simulink model "pendulo_rueda_lazo_cerrado_LQR"  (R2021b)
settings: Solver=ode5  StartTime=0.0  StopTime=30  FixedStep=0.01  RelTol=1e-3  EnableMultiTasking=on
values from neighbouring files (symbols this model uses):
  A = [0, 1, 0, 0;b4, 0, 0, b5;0, 0, 0, 1;b7, 0, 0, b8]    [Diseno_controlador_LQR.m]
  B = [0;b6;0;b9]    [Diseno_controlador_LQR.m]
  C = [1,0,0,0;0,0,1,0]    [Diseno_controlador_LQR.m]
  K_LQR = lqr(A,B,Q,r)    [Diseno_controlador_LQR.m]
undefined symbols (not defined in the file or in its folder): Ke_uno, National_Instruments, PCIe
libraries: sldrtlib x5
Description:
  | Real-Time Van der Pol Simulation
  | 
  | The example model "sldrtex_vdp" shows a real-time version of the Simulink(R) Van der Pol
  | simulation model. This model does not need any external signals, so it does
  | not need any data acquisition hardware or driver. This makes the model ideal
  | for the first experiments with Simulink Desktop Real-Time(TM), without need to
  | worry about proper I/O hardware configuration.
  | 
  | How to run this model in Normal Mode:
  | 
  | 1) Double-click the orange button to switch to Normal Mode if needed.
  | 2) Start the real-time execution using Simulation->Run.
  | 3) Observe any missed ticks on the Missed Ticks scope.
  | 
  | How to run this model in External Mode:
  | 
  | 1) Double-click the orange button to switch to External Mode if needed.
  | 2) Start the real-time execution using Simulation->Run. The model will automatically
  |    build, connect to Simulink in External Mode and start.
  | 3) Missed ticks will be always zero.
settings Model: ExtModeTrigDuration=100001  ExtModeLogAll=off  Creator=The MathWorks, Inc.  LastModifiedBy=USUARIO
settings SolverCC: AlgebraicLoopSolver=TrustRegion
settings DataIOCC: LimitDataPoints=on  SaveFormat=Array  ReturnWorkspaceOutputs=off  SignalLoggingName=logsOut
settings OptimizationCC: ExpressionDepthLimit=2147483647  InitFltsAndDblsToZero=on  EfficientMapNaN2IntZero=off  LifeSpan=inf
settings DebuggingCC: UnderspecifiedInitializationDetection=Classic  MergeDetectMultiDrivingBlocksExec=none  SignalResolutionControl=TryResolveAllWithWarning  FcnCallInpInsideContextMsg=warning  AllowSymbolicDim=off  StateNameClashWarn=warning  SymbolicDimsDataTypeCodeGenerationDiagnostic=none  SFUnexpectedBacktrackingDiag=warning  SFNoUnconditionalDefaultTransitionDiag=warning  SFExecutionAtInitializationDiag=none  SFMachineParentedDataDiag=warning  ArithmeticOperatorsInVariantConditions=warning
settings HardwareCC: TargetBitPerLong=64  TargetBitPerPointer=64  TargetBitPerSizeT=64  TargetBitPerPtrDiffT=64  TargetIntDivRoundTo=Zero  TargetEndianess=LittleEndian  TargetWordSize=64  TargetHWDeviceType=Intel->x86-64
settings ModelReferenceCC: PropagateSignalLabelsOutOfModel=off
settings SFSimCC: SimUseLocalCustomCode=off
settings RTWCC: Description=Simulink Desktop Real-Time  SystemTargetFile=sldrt.tlc  TemplateMakefile=sldrt.tmf  RTWUseLocalCustomCode=off  RTWCompilerOptimization=on
settings CodeAppCC: MaxIdLength=95  StateflowObjectComments=on
settings SimulinkDesktopRealTimeCC: TargetPreCompLibLocation=C:\Program Files\MATLAB\R2021b\toolbox\sldrt\lib\win64  TargetLangStandard=C89/C90 (ANSI)  SupportVariableSizeSignals=off
settings ConfigComp: CovMetricSettings=dw  CovSaveCumulativeToWorkspaceVar=on  CovSaveSingleToWorkspaceVar=on  CovExternalEMLEnable=off  CovSFcnEnable=off

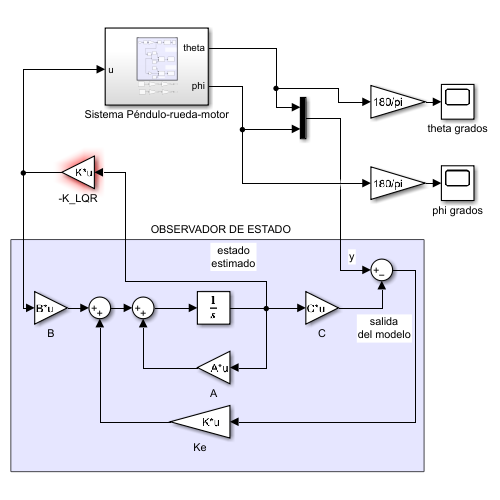
[thumbnail: Simulink's stored preview of the top-level diagram]
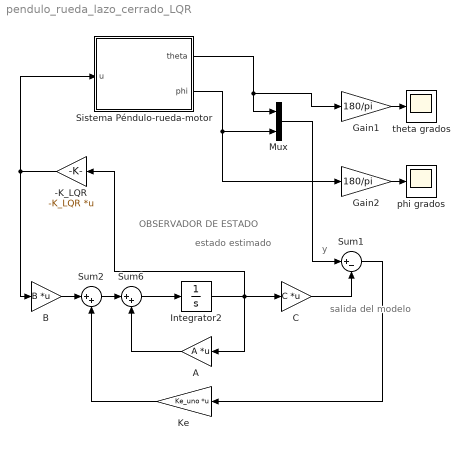
== system pendulo_rueda_lazo_cerrado_LQR ==
  note: OBSERVADOR DE ESTADO
  note: estado
      | estimado
  note: salida
      | del modelo
  note: y
  -K_LQR : Gain  Gain=-K_LQR  Multiplication=Matrix(K*u)
  A : Gain  Gain=A  Multiplication=Matrix(K*u)
  B : Gain  Gain=B  Multiplication=Matrix(K*u)
  C : Gain  Gain=C  Multiplication=Matrix(K*u)
  Gain1 : Gain  Gain=180/pi
  Gain2 : Gain  Gain=180/pi
  Integrator2 : Integrator
  Ke : Gain  Gain=Ke_uno  Multiplication=Matrix(K*u)
  Mux : Mux  Inputs=2
  Sistema Péndulo-rueda-motor : Subsystem
  Sum1 : Sum  Inputs=|+-
  Sum2 : Sum  Inputs=|++
  Sum6 : Sum  Inputs=|++
  phi grados : Scope
  theta grados : Scope
  wires:
  Integrator2/1 -> -K_LQR/1, A/1, C/1
  Sum6/1 -> Integrator2/1
  C/1 -> Sum1/2
  Sum1/1 -> Ke/1
  A/1 -> Sum6/2
  Ke/1 -> Sum2/2
  Sum2/1 -> Sum6/1
  B/1 -> Sum2/1
  Mux/1 -> Sum1/1
  Sistema Péndulo-rueda-motor/2(phi) -> Gain2/1, Mux/2
  Sistema Péndulo-rueda-motor/1(theta) -> Gain1/1, Mux/1
  Gain1/1 -> theta grados/1
  Gain2/1 -> phi grados/1
  -K_LQR/1 -> Sistema Péndulo-rueda-motor/1(u), B/1

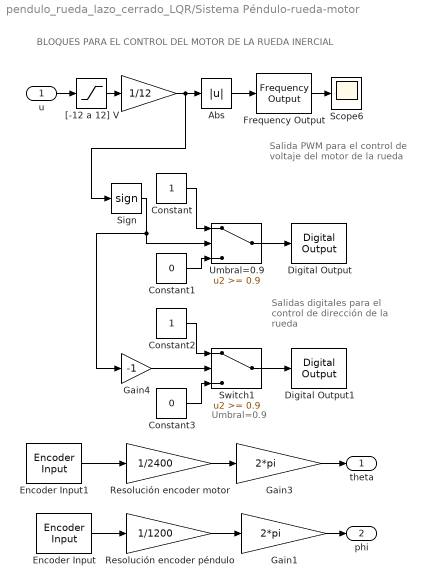
== system pendulo_rueda_lazo_cerrado_LQR/Sistema Péndulo-rueda-motor ==
  note: BLOQUES PARA EL CONTROL DEL MOTOR DE LA RUEDA INERCIAL
  note: Umbral=0.9
  note: Salida PWM para el
      |  control de voltaje del
      |   motor de la rueda
  note: Salidas digitales
      |    para el control de
      | dirección de la rueda
  u : Inport
  "   " : Gain  Gain=1/12
  "      Resolución encoder péndulo" : Gain  Gain=1/1200
  Abs : Abs
  Constant : Constant
  Constant1 : Constant  Value=0
  Constant2 : Constant
  Constant3 : Constant  Value=0
  Digital Output : sldrtlib/Digital Output  SampleTime=0.01  MaxMissedTicks=100  ShowMissedTicks=off  YieldWhenWaiting=off  DrvName=National_Instruments/PCIe-6321  DrvAddress=4294967295  DrvOptions=[0 3 16384 0 2 3 2]  Channels=1  BitMode=1  InitialValue=[]  FinalValue=[]
      settings: AttributesFormatString=National Instruments\nPCIe-6321 [auto]  SourceProductBaseCode=WT
  Digital Output1 : sldrtlib/Digital Output  SampleTime=0.01  MaxMissedTicks=100  ShowMissedTicks=off  YieldWhenWaiting=off  DrvName=National_Instruments/PCIe-6321  DrvAddress=4294967295  DrvOptions=[0 3 16384 0 2 3 2]  Channels=2  BitMode=1  InitialValue=[]  FinalValue=[]
      settings: AttributesFormatString=National Instruments\nPCIe-6321 [auto]  SourceProductBaseCode=WT
  Encoder Input : sldrtlib/Encoder Input  SampleTime=0.01  MaxMissedTicks=100  ShowMissedTicks=off  YieldWhenWaiting=off  DrvName=National_Instruments/PCIe-6321  DrvAddress=4294967295  DrvOptions=[0 3 16384 0 2 3 2]  Channels=4  QuadMode=3  IndexPulse=2  InputFilter=Inf  DataType=1
      settings: AttributesFormatString=National Instruments\nPCIe-6321 [auto]
  Encoder Input1 : sldrtlib/Encoder Input  SampleTime=0.01  MaxMissedTicks=100  ShowMissedTicks=off  YieldWhenWaiting=off  DrvName=National_Instruments/PCIe-6321  DrvAddress=4294967295  DrvOptions=[0 3 16384 0 2 3 2]  Channels=2  QuadMode=3  IndexPulse=1  InputFilter=Inf  DataType=1
      settings: AttributesFormatString=National Instruments\nPCIe-6321 [auto]
  Frequency Output : sldrtlib/Frequency Output  SampleTime=0.01  MaxMissedTicks=100  ShowMissedTicks=on  YieldWhenWaiting=off  DrvName=National_Instruments/PCIe-6321  DrvAddress=4294967295  DrvOptions=[0 3 16384 0 2 3 2]  Channels=3  FrequencySource=1  Frequency=500  FrequencyFinalValue=[]  DutySource=2  Duty=0  DutyFinalValue=0
      settings: AttributesFormatString=National Instruments\nPCIe-6321 [auto]  SourceProductBaseCode=WT
  Gain1 : Gain  Gain=2*pi
  Gain3 : Gain  Gain=2*pi
  Gain4 : Gain  Gain=-1
  Resolución encoder motor : Gain  Gain=1/2400
  Scope6 : Scope
  Sign : Signum
  Switch1 : Switch  Threshold=0.9
  Umbral=0.9 : Switch  Threshold=0.9
  "[-12 a 12] V" : Saturate  UpperLimit=12  LowerLimit=-12
  theta : Outport
  phi : Outport  Port=2
  wires:
  u/1 -> "[-12 a 12] V"/1
  Frequency Output/1 -> Scope6/1
  Abs/1 -> Frequency Output/1
  Switch1/1 -> Digital Output1/1
  Umbral=0.9/1 -> Digital Output/1
  Encoder Input/1 -> "      Resolución encoder péndulo"/1
  "      Resolución encoder péndulo"/1 -> Gain1/1
  Resolución encoder motor/1 -> Gain3/1
  Encoder Input1/1 -> Resolución encoder motor/1
  Gain3/1 -> theta/1
  Gain1/1 -> phi/1
  Constant3/1 -> Switch1/3
  Constant2/1 -> Switch1/1
  Sign/1 -> Gain4/1, Umbral=0.9/2
  "[-12 a 12] V"/1 -> "   "/1
  Constant1/1 -> Umbral=0.9/3
  Constant/1 -> Umbral=0.9/1
  "   "/1 -> Sign/1, Abs/1
  Gain4/1 -> Switch1/2
